simulink model "DC_tuning"  (R2023b)
settings: Solver=VariableStepAuto  StartTime=0.0  StopTime=200  RelTol=1e-3
values from neighbouring files (symbols this model uses):
  CM = 2.909*10^-5    (= 2.909e-05)    [dcdata.m]
  Jm = 6.24*10^-4    (= 0.000624)    [dcdata.m]
  Kb = 1.7629*10^-2    (= 0.017629)    [dcdata.m]
  Kt = 1.7629*10^-2    (= 0.017629)    [dcdata.m]
  La = 0.28    [dcdata.m]
  Ra = 0.22680    (= 0.2268)    [dcdata.m]
  Trat = Ia*Kt    (= 0.158661)    [dcdata.m]
  wm = 564.9    [dcdata.m]
libraries: SignalEditorBlockLib x1, slpidlib x1
settings Model: Creator=Matth  LastModifiedBy=chris

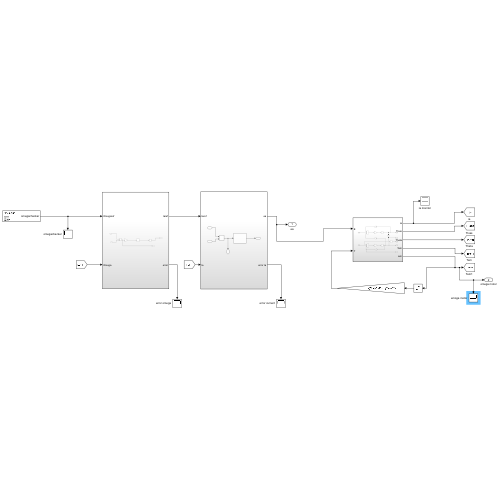
[thumbnail: Simulink's stored preview of the top-level diagram]
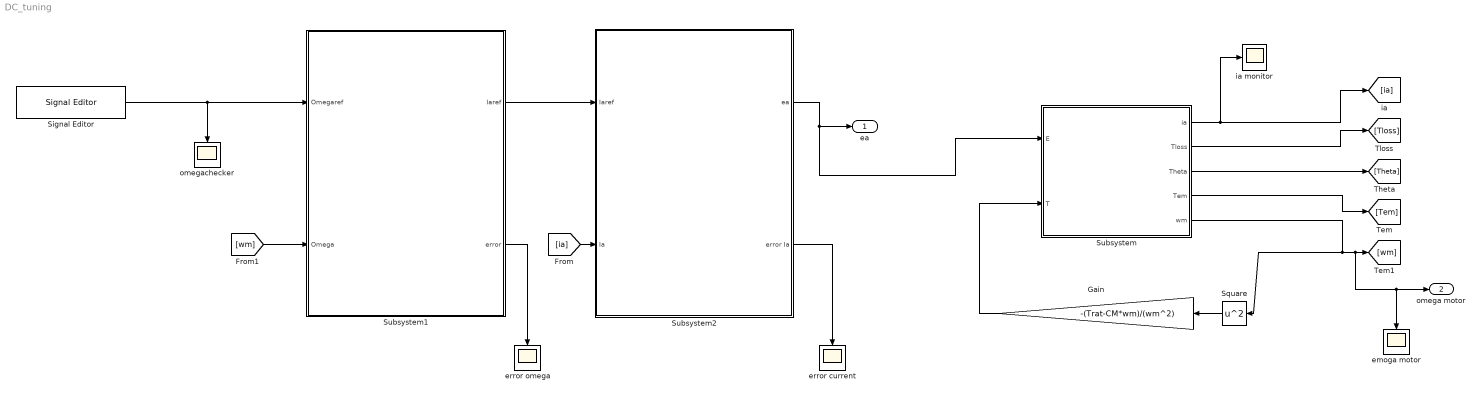
== system DC_tuning ==
  Gain : Gain  Gain=-(Trat-CM*wm)/(wm^2)
  Signal Editor : SignalEditorBlockLib/Signal Editor  FileName=C:\Users\chris\Documents\master\mechatronics in MT\simulations\omegachecker.mat  ActiveScenario=Scenario  ActiveSignal=omegachecker  IsBus=off  OutputBusObjectStr=Bus: BusObject  SampleTime=0  OutputAfterFinalValue=Setting to zero  Unit=inherit  PreserveSignalName=on  ApplySigPropsToAllScenarios=on  ApplySigPropsToAllSignals=on
  Square : Math  Operator=square
  Subsystem : Subsystem
  Subsystem1 : Subsystem
  Subsystem2 : Subsystem
  emoga motor : Scope
  error current : Scope
  error omega : Scope
  ia monitor : Scope
  omegachecker : Scope
  ea : Outport
  omega motor : Outport  Port=2
  wires:
  Subsystem/2(Tloss) -> [Tloss]
  [ia] -> Subsystem2/2(Ia)
  Subsystem/3(Theta) -> [Theta]
  Square/1 -> Gain/1
  Subsystem1/1(Iaref) -> Subsystem2/1(Iaref)
  Gain/1 -> Subsystem/2(T)
  Subsystem/5(wm) -> emoga motor/1, omega motor/1, [wm], Square/1
  Subsystem2/1(ea) -> Subsystem/1(E), ea/1
  Subsystem/1(ia) -> ia monitor/1, [ia]
  Subsystem/4(Tem) -> [Tem]
  Subsystem1/2(error) -> error omega/1
  [wm] -> Subsystem1/2(Omega)
  Subsystem2/2(error Ia) -> error current/1
  Signal Editor/1 -> omegachecker/1, Subsystem1/1(Omegaref)

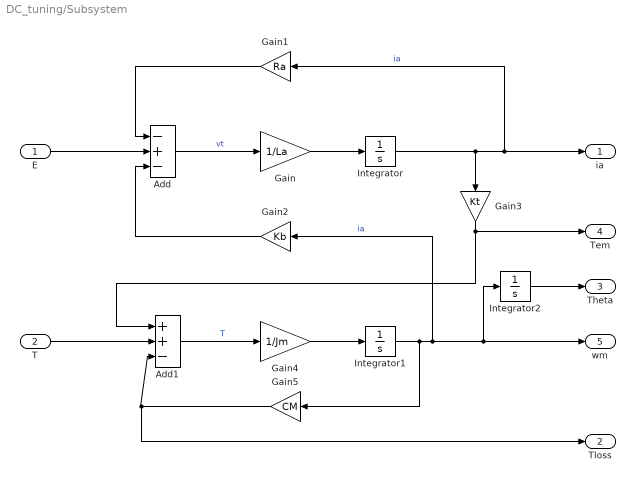
== system DC_tuning/Subsystem ==
  E : Inport
  T : Inport  Port=2
  Add : Sum  Inputs=-+-
  Add1 : Sum  Inputs=++-
  Gain : Gain  Gain=1/La
  Gain1 : Gain  Gain=Ra
  Gain2 : Gain  Gain=Kb
  Gain3 : Gain  Gain=Kt
  Gain4 : Gain  Gain=1/Jm
  Gain5 : Gain  Gain=CM
  Integrator : Integrator
  Integrator1 : Integrator
  Integrator2 : Integrator
  ia : Outport
  Tloss : Outport  Port=2
  Theta : Outport  Port=3
  Tem : Outport  Port=4
  wm : Outport  Port=5
  wires:
  Gain2/1 -> Add/3
  Gain/1 -> Integrator/1
  Integrator1/1 -> wm/1, Integrator2/1, Gain2/1, Gain5/1  "ia"
  Add1/1 -> Gain4/1  "T"
  Add/1 -> Gain/1  "vt"
  Gain1/1 -> Add/1
  Gain4/1 -> Integrator1/1
  Integrator/1 -> ia/1, Gain1/1, Gain3/1  "ia"
  Gain3/1 -> Add1/1, Tem/1
  Gain5/1 -> Tloss/1, Add1/3
  E/1 -> Add/2
  T/1 -> Add1/2
  Integrator2/1 -> Theta/1

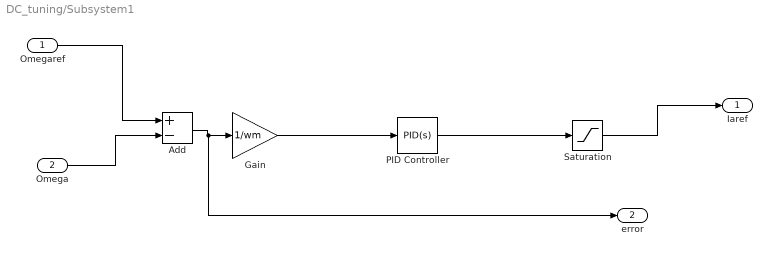
== system DC_tuning/Subsystem1 ==
  Omegaref : Inport
  Omega : Inport  Port=2
  Add : Sum  Inputs=+-
  Gain : Gain  Gain=1/wm
  PID Controller : slpidlib/PID Controller  Controller=PID  Form=Ideal  TimeDomain=Continuous-time  UseExternalTs=off  SampleTime=-1  IntegratorMethod=Forward Euler  FilterMethod=Forward Euler  ControllerParametersSource=internal  P=405.629755501979  I=0.388928592826706  UseKiTs=off  D=0.571282734671085  N=7618.85317361069  UseFilter=on  TunerSelectOption=Transfer Function Based (PID Tuner App)  InitialConditionSource=internal  InitialConditionForIntegrator=0  InitialConditionForFilter=0  DifferentiatorICPrevScaledInput=0  ExternalReset=none  TrackingMode=off  Kt=1  LimitOutput=off  SatLimitsSource=internal  UpperSaturationLimit=inf  LowerSaturationLimit=-inf  LinearizeAsGain=on  AntiWindupMode=none  Kb=1  LimitIntegrator=off  UpperIntegratorSaturationLimit=inf  LowerIntegratorSaturationLimit=-inf  POutMin=[]  POutMax=[]  IOutMin=[]  IOutMax=[]  DOutMin=[]  DOutMax=[]  NOutMin=[]  NOutMax=[]  SumOutMin=[]  SumOutMax=[]  SaturationOutMin=[]  SaturationOutMax=[]  PParamMin=[]  PParamMax=[]  IParamMin=[]  IParamMax=[]  DParamMin=[]  DParamMax=[]  NParamMin=[]  NParamMax=[]  KbParamMin=[]  KbParamMax=[]  KtParamMin=[]  KtParamMax=[]  KbOutMin=[]  KbOutMax=[]  KtOutMin=[]  KtOutMax=[]  IntegratorOutMin=[]  IntegratorOutMax=[]  FilterOutMin=[]  FilterOutMax=[]  SumI1OutMin=[]  SumI1OutMax=[]  SumI2OutMin=[]  SumI2OutMax=[]  SumI3OutMin=[]  SumI3OutMax=[]  SumI4OutMin=[]  SumI4OutMax=[]  SumDOutMin=[]  SumDOutMax=[]  DifferentiatorOutMin=[]  DifferentiatorOutMax=[]  FilterDiffOutCoefMin=[]  FilterDiffOutCoefMax=[]  ReciprocalOutMin=[]  ReciprocalOutMax=[]  SumDenOutMin=[]  SumDenOutMax=[]  SumNumOutMin=[]  SumNumOutMax=[]  DivideOutMin=[]  DivideOutMax=[]  UdiffTsProdOutMin=[]  UdiffTsProdOutMax=[]  NTsProdOutMin=[]  NTsProdOutMax=[]  UintegralTsProdOutMin=[]  UintegralTsProdOutMax=[]  UngainTsProdOutMin=[]  UngainTsProdOutMax=[]  ClampingZeroOutDataTypeStr=Inherit: Inherit via back propagation  ClampingZeroOutMin=[]  ClampingZeroOutMax=[]  FilterDenConstantOutDataTypeStr=Inherit: Inherit via back propagation  FilterDenConstantOutMin=[]  FilterDenConstantOutMax=[]  PCopyOutDataTypeStr=Inherit: Inherit via back propagation  PCopyOutMin=[]  PCopyOutMax=[]  NCopyOutDataTypeStr=Inherit: Inherit via back propagation  NCopyOutMin=[]  NCopyOutMax=[]  IntegratorContinuousStateAttributes=''  IntegratorStateMustResolveToSignalObject=off  IntegratorRTWStateStorageClass=Auto  FilterContinuousStateAttributes=''  FilterStateMustResolveToSignalObject=off  FilterRTWStateStorageClass=Auto  ParallelPVariant=Passthrough  IdealPVariant=InternalParameters  IVariant=InternalParameters  DVariant=InternalParameters  IntegratorVariant=Continuous  SatVariant=Disabled  AWVariant=Passthrough  PCopyVariant=Disabled  TRVariant=Disabled  FdbkBlocksVariant=Forward  IdealPFdbkVariant=Disabled  SatFdbkVariant=Disabled  DerivativeFilterVariant=ContFilter  NVariant=InternalParameters  NCopyVariant=Disabled  FilterICVariant=InternalICsFilter  IntegratorICVariant=InternalICs  ExternalResetVariant=Disabled  TRSumVariant=Passthrough  SumFdbkVariant=Disabled  SumVariant=Sum_PID  TsampFilterVariant=InternalTs  TsampNgainVariant=Passthrough  TsampIntegralVariant=Disabled_SignalSpec  ExternalSaturationOutDataTypeStr=Inherit: Same as second input
  Saturation : Saturate  UpperLimit=9  LowerLimit=-9
  Iaref : Outport
  error : Outport  Port=2
  wires:
  Omegaref/1 -> Add/1
  Omega/1 -> Add/2
  Add/1 -> error/1, Gain/1
  Gain/1 -> PID Controller/1
  Saturation/1 -> Iaref/1
  PID Controller/1 -> Saturation/1

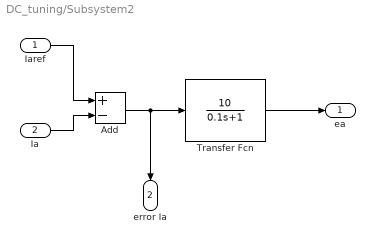
== system DC_tuning/Subsystem2 ==
  Iaref : Inport
  Ia : Inport  Port=2
  Add : Sum  Inputs=+-
  Transfer Fcn : TransferFcn  Numerator=[10]  Denominator=[0.1 1]
  ea : Outport
  error Ia : Outport  Port=2
  wires:
  Iaref/1 -> Add/1
  Ia/1 -> Add/2
  Add/1 -> error Ia/1, Transfer Fcn/1
  Transfer Fcn/1 -> ea/1
